simulink model "double_pend_natural"  (R2021a)
settings: Solver=VariableStepAuto  StartTime=0.0  StopTime=40  RelTol=1e-7
values from neighbouring files (symbols this model uses):
  I1 = 0.1*(0.1^2+0.0254^2)/12+0.2*l1^2/2+0.2*R1^2    (= 0.0504180596667)    [rundoublesim.m]
  I2 = 0.1*(0.1^2+0.0254^2)/12    (= 8.87096666667e-05)    [rundoublesim.m]
  l1 = 0.459    [rundoublesim.m]
  m1 = 0.3    [rundoublesim.m]
  m2 = 0.1    [rundoublesim.m]
  R1 = (0.1*l1/2+l1*0.2)/0.3    (= 0.3825)    [rundoublesim.m]
  R2 = 0.459/2    (= 0.2295)    [rundoublesim.m]
settings Model: Creator=natha  LastModifiedBy=natha

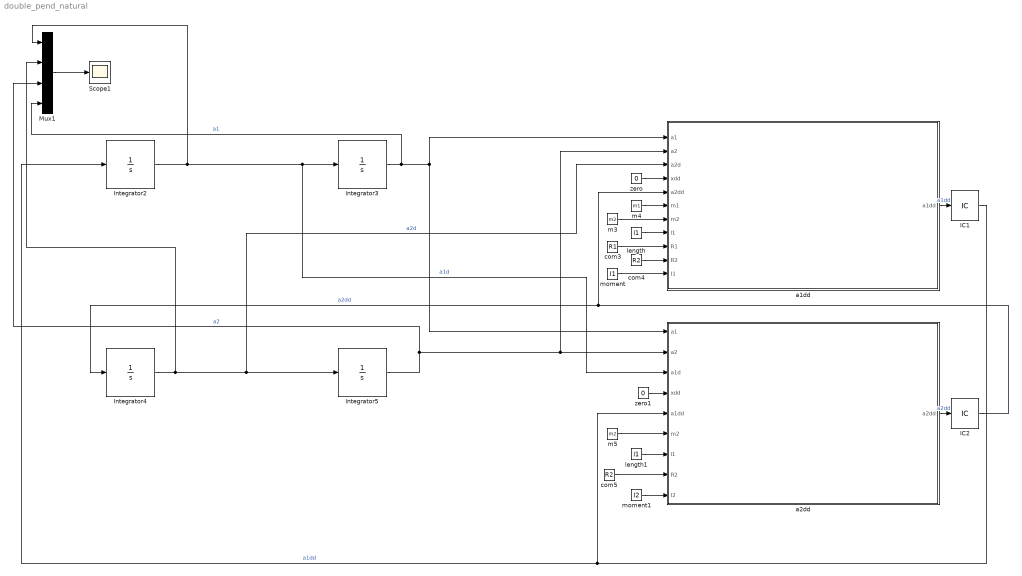
== system double_pend_natural ==
  IC1 : InitialCondition  Value=0
  IC2 : InitialCondition  Value=0
  Integrator2 : Integrator
  Integrator3 : Integrator  InitialCondition=3.14
  Integrator4 : Integrator
  Integrator5 : Integrator  InitialCondition=3.142/2
  Mux1 : Mux
  Scope1 : Scope
  a1dd : MATLAB Function  TreatAsAtomicUnit=on
  a2dd : MATLAB Function  TreatAsAtomicUnit=on
  com3 : Constant  Value=R1
  com4 : Constant  Value=R2
  com5 : Constant  Value=R2
  length : Constant  Value=l1
  length1 : Constant  Value=l1
  m3 : Constant  Value=m2
  m4 : Constant  Value=m1
  m5 : Constant  Value=m2
  moment : Constant  Value=I1
  moment1 : Constant  Value=I2
  zero : Constant  Value=0
  zero1 : Constant  Value=0
  wires:
  com4/1 -> a1dd/10(R2)
  com3/1 -> a1dd/9(R1)
  length/1 -> a1dd/8(l1)
  m3/1 -> a1dd/7(m2)
  m4/1 -> a1dd/6(m1)
  moment/1 -> a1dd/11(I1)
  m5/1 -> a2dd/6(m2)
  length1/1 -> a2dd/7(l1)
  com5/1 -> a2dd/8(R2)
  moment1/1 -> a2dd/9(I2)
  IC2/1 -> a1dd/5(a2dd), Integrator4/1  "a2dd"
  Integrator4/1 -> Mux1/2, a1dd/3(a2d), Integrator5/1  "a2d"
  Integrator5/1 -> Mux1/3, a1dd/2(a2), a2dd/2(a2)  "a2"
  IC1/1 -> Integrator2/1, a2dd/5(a1dd)  "a1dd"
  Integrator2/1 -> Mux1/1, a2dd/3(a1d), Integrator3/1  "a1d"
  Integrator3/1 -> Mux1/4, a2dd/1(a1), a1dd/1(a1)  "a1"
  Mux1/1 -> Scope1/1
  a1dd/1(a1dd) -> IC1/1  "a1dd"
  a2dd/1(a2dd) -> IC2/1  "a2dd"
  zero/1 -> a1dd/4(xdd)
  zero1/1 -> a2dd/4(xdd)

== matlab function double_pend_natural/a1dd ==
  data: a1 input; a1dd output; a2 input; a2d input; xdd input; a2dd input; m1 input; m2 input; l1 input; R1 input; R2 input; I1 input
function a1dd  = a1doubledot(a1,a2,a2d,xdd,a2dd,m1,m2,l1,R1,R2,I1)
%calculates the angle 1 double dot term givin the other variables
    s1 = sin(a1);
    s2 = sin(a2);
    c1 = cos(a1);
    c2 = cos(a2);
    sig2=a2d^2;
    sig3=s1^2;
    sig4=c1^2;
    sig5 = xdd;
    sig6 = a2dd;
    g=9.806;
    denom = -(I1+R1^2*m1*sig4+R1^2*m1*sig3+l1^2*m2*sig4+l1^2*m2*sig3);
    num = R1*m1*c1*sig5+ l1*m2*c1*sig5 + R1*g*m1*s1 + g*l1*m2*s1 - R2*l1*m2*c1*s2*sig2 + R2*l1*m2*c2*s1*sig2 + R2*l1*m2*c1*c2*sig6 + R2*l1*m2*s1*s2*sig6;
    a1dd=num/denom;
end

== matlab function double_pend_natural/a2dd ==
  data: a1 input; a2dd output; a2 input; a1d input; xdd input; a1dd input; m2 input; l1 input; R2 input; I2 input
function a2dd  = a2doubledot(a1,a2,a1d,xdd,a1dd,m2,l1,R2,I2)
%calculates the angle 2 double dot term givin the other variables
    s1 = sin(a1);
    s2 = sin(a2);
    c1 = cos(a1);
    c2 = cos(a2);
    sig2=a1d^2;
    sig3=a1dd;
    g=9.806;
    denom =-(I2+R2^2*m2*c2^2+R2^2*m2*s2^2);
    num = R2*m2*c2*xdd+R2*g*m2*s2+R2*l1*m2*c1*s2*sig2-R2*l1*m2*c2*s1*sig2+R2*l1*m2*c1*c2*sig3+R2*l1*m2*s1*s2*sig3;
    a2dd=num/denom;
end
